simulink model "matched_filter_offset_estimation_correction"  (R2014b)
settings: Solver=FixedStepDiscrete  SolverMode=SingleTasking  StartTime=0.0  StopTime=run_time  RelTol=1e-3
PreLoadFcn:
  | %%%%%%%%%%%%%%%%%%%%%%%%%%%%%%%%%%%%%%%%%%%%%%%%%%%%%%%%%%%%%%%%%%%%%%%%%%%
  | % check to see if Simulink library folder is missing from the MATLAB path %
  | %%%%%%%%%%%%%%%%%%%%%%%%%%%%%%%%%%%%%%%%%%%%%%%%%%%%%%%%%%%%%%%%%%%%%%%%%%%
  | if isempty(strfind(path, 'rtlsdr_book_library'))
  | 
  |     % create error window
  |     fig_error = figure(...
  |         'Name', 'Error: RTL-SDR Book Library',...
  |         'Toolbar','none',...
  |         'MenuBar','none',...
  |         'NumberTitle','off',...
  |         'Resize','off',...
  |         'WindowStyle','modal');
  |     fig_error.Position(3) = 600;
  |     fig_error.Position(4) = 150;
  |     fig_axes = axes(...
  |         'Parent',fig_error,...
  |         'Position',[0,0,1,1],...
  |         'visible','off');
  |     % error message
  |     t_title = text(.05,.8,...
  |         'MISSING DIRECTORIES',...
  |         'FontSize',11.5);
  |     t_body = text(.075,.6,...
  |         [{'Simulink cannot find the  \it{<root>}\rm / \it{rtlsdr\_book\_library}\rm  folder in the \it{MATLAB Path}\rm.'},...
  |         {'Please set the MATLAB path following the instructions given in Exercise 2.4.'}],...
  |         'FontSize',10.5);
  |     % buttons
  |     btn_path = uicontrol(...
  |         'Parent',fig_error,...
  |         'String','Set Path Now',...
  |         'FontSize',10,...
  |         'Callback', 'pathtool; close(fig_error);',...
  |         'Position', [fig_error.Position(3)/2-210, 30, 200, 30]);
  |     btn_abort = uicontrol(...
  |         'Parent',fig_error,...
  |         'String','No thanks',...
  |         'FontSize',10,...
  |         'Callback', 'close(fig_error); abort=1;',...
  |         'Position', [fig_error.Position(3)/2+10, 30, 200, 30]);
  | 
  |     % pause to allow user to interact with error box
  |     uiwait(fig_error);
  | 
  |     % abort simulation
  |     try
  |         if abort==1
  |             set_param(gcs, 'SimulationCommand', 'stop');
  |         end
  |     end
  | 
  |     % if user has set path, allow diagram to be updated
  |     if ~exist('abort','var')
  |         % create error window
  |         fig_update = figure(...
  |             'Name', 'Update Diagram',...
  |             'Toolbar','none',...
  |             'MenuBar','none',...
  |             'NumberTitle','off',...
  |             'Resize','off');
  |         fig_update.Position(3) = 400;
  |         fig_update.Position(4) = 120;
  |         fig_axes = axes(...
  |             'Parent',fig_update,...
  |             'Position',[0,0,1,1],...
  |             'visible','off');
  |         % instruction message
  |         t_body = text(.075,.7,...
  |             'Once you have set the path, update the block diagram',...
  |             'FontSize',10.5);
  |         % button
  |         btn_update = uicontrol(...
  |             'Parent',fig_update,...
  |             'String','Update Block Diagram',...
  |             'FontSize',10,...
  |             'Callback', 'set_param(gcs,''SimulationCommand'',''update''); close(gcf)',...
  |             'Position', [fig_update.Position(3)/2-100, 30, 200, 30]);
  |     end
  | 
  |     % clear error components
  |     clear('fig_error','fig_update','fig_axes','t_title','t_body','btn_path','btn_abort','btn_update','abort');
  | 
  | end
  | %%%%%%%%%%%%%%%%%%%%%%%%%%%%%%%%%%%%%%%%%%%%%%%%%%%%%%%%%%%%%%%%%%%%%%%%%%%
  | 
  | 
  | % create default variable for running model
  | run_time = 7.3;
undefined symbols (not defined in the file): rec
libraries: simulink x5, rtlsdr_book_library x2, commutil2 x2, commdigbbndpm3 x2, dspmtrx3 x1
CloseFcn:
  | closefcn_model;
Description:
  | Software, Simulation Examples and Design Exercises Licence Agreement
  | 
  | This license agreement refers to the simulation examples, design exercises and files,
  | and associated software MATLAB and Simulink resources that accompany the book:
  | 
  |      Title: Software Defined Radio using MATLAB & Simulink and the RTL-SDR
  |      Published by Strathclyde Academic Media, 2015
  |      Authored by Robert W. Stewart, Kenneth W. Barlee, Dale S.W. Atkinson,
  |      and Louise H. Crockett
  | 
  | and made available as a download from, www.desktopSDR.com or variously acquired
  | by other means such as via USB storage, cloud storage, disk or any other electronic
  | or optical or magnetic storage mechanism. These files and associated software may
  | be used subject to the terms of agreement of the conditions below:
  | 
  |     Copyright © 2015 Robert W. Stewart, Kenneth W. Barlee, Dale S.W. Atkinson,
  |     and Louise H. Crockett
  |     All rights reserved.
  | 
  | Redistribution and use in source and binary forms, with or without modification, are
  | permitted provided that the following conditions are met:
  | 
  |    1.  Redistributions of source code must retain the above copyright notice, this list of
  |         conditions and the following disclaimer.
  | 
  |    2.  Redistributions in binary form must reproduce the above copyright notice, this
  |         list of conditions and the following disclaimer in the documentation and/or other
  |         materials provided with the distribution.
  | 
  |    3.  Neither the name of the copyright holder nor the names of its contributors may
  |         be used to endorse or promote products derived from this software without
  |         specific prior written permission.
  | 
  |    4.  In all cases, the software is, and all modifications and derivatives of the
  |         software shall be, licensed to you solely for use in conjunction with The
  |         MathWorks, Inc. products and service offerings.
  | 
  | THIS SOFTWARE IS PROVIDED BY THE COPYRIGHT HOLDERS AND CONTRIBUTORS
  | "AS IS" AND ANY EXPRESS OR IMPLIED WARRANTIES, INCLUDING, BUT NOT LIMITED
  | TO, THE IMPLIED WARRANTIES OF MERCHANTABILITY AND FITNESS FOR A
  | PARTICULAR PURPOSE ARE DISCLAIMED. IN NO EVENT SHALL THE COPYRIGHT
  | HOLDER OR CONTRIBUTORS BE LIABLE FOR ANY DIRECT, INDIRECT, INCIDENTAL,
  | SPECIAL, EXEMPLARY, OR CONSEQUENTIAL DAMAGES (INCLUDING, BUT NOT
  | LIMITED TO, PROCUREMENT OF SUBSTITUTE GOODS OR SERVICES; LOSS OF USE,
  | DATA, OR PROFITS; OR BUSINESS INTERRUPTION) HOWEVER CAUSED AND ON ANY
  | THEORY OF LIABILITY, WHETHER IN CONTRACT, STRICT LIABILITY, OR TORT
  | (INCLUDING NEGLIGENCE OR OTHERWISE) ARISING IN ANY WAY OUT OF THE USE
  | OF THIS SOFTWARE, EVEN IF ADVISED OF THE POSSIBILITY OF SUCH DAMAGE.
  | 
  | 
  | Audio Tracks used in Simulations Examples and Design Exercises
  | 
  | The music and vocal files used within the Examples files and software within the book
  | were variously written, arranged, performed, recorded and produced by Garrey Rice,
  | Adam Struth, Jamie Struth, Iain Thistlethwaite and also Marshall Craigmyle who
  | collectively, and individually where appropriate, assert and retain all of their copyright,
  | performance and artistic rights. Permission to use and reproduce this music is
  | granted for all purposes associated with MATLAB and Simulink software and the
  | simulation examples and design exercises files that accompany this book. Requests to
  | use the music for any other purpose should be directed to: info@desktopSDR.com.
  | For information on music track names, full credits, and links to the musicians please
  | refer to www.desktopSDR.com/more/audio.
settings Model: Creator=desktopSDR Team  LastModifiedBy=desktopSDR Team
settings DataIOCC: LimitDataPoints=off  SaveOutput=off  SignalLogging=off  SaveTime=off

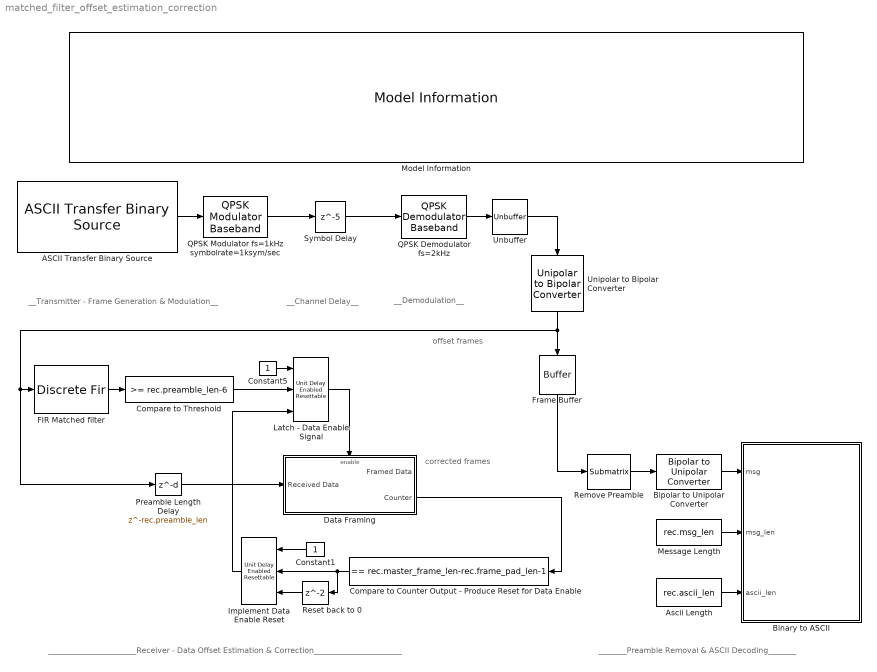
== system matched_filter_offset_estimation_correction ==
  note: corrected frames
  note: offset frames
  note: __Transmitter - Frame Generation & Modulation__
  note: __Channel Delay__
  note: __Demodulation__
  note: ______________________Receiver - Data Offset Estimation & Correction______________________
  note: _______Preamble Removal & ASCII Decoding_______
  "  ASCII Transfer Binary Source" : rtlsdr_book_library/Data Comms Sources and Sinks/  ASCII Transfer Binary Source  msg_tx=Hello World!  fs=2e3
  Ascii Length : Constant  Value=rec.ascii_len  VectorParams1D=off  OutDataTypeStr=single  FramePeriod=4096/240e3
  Binary to ASCII : MATLAB Function  TreatAsAtomicUnit=on
      mask init:
      | %% FIGURE SETUP        
      | %figure;
      | 
      | % resize
      | %window_x = 500;
      | %window_y = 500;
      | %window_width = 500;
      | %window_height = 110;
      | %set(gcf, 'Position', [window_x window_y window_width window_height]);
      | %set(gcf, 'menubar', 'none');
  Bipolar to Unipolar Converter : commutil2/Bipolar to Unipolar Converter  M=2  polarity=Positive  dataType=Inherit via internal rule
  Compare to Counter Output - Produce Reset for Data Enable : simulink/Logic and Bit Operations/Compare To Constant  relop===  const=rec.master_frame_len-rec.frame_pad_len-1  OutDataTypeStr=boolean
  Compare to Threshold : simulink/Logic and Bit Operations/Compare To Constant  relop=>=  const=rec.preamble_len-6  OutDataTypeStr=boolean
  Constant1 : Constant
  Constant5 : Constant
  Data Framing : Subsystem
  FIR Matched filter : DiscreteFir  Coefficients=rec.filter_coeff  InputProcessing=Columns as channels (frame based)
  Frame Buffer : Buffer  N=rec.master_frame_len  TreatMby1Signals=One channel
  Implement Data Enable Reset : simulink/Additional Math & Discrete/Additional Discrete/Unit Delay Enabled Resettable  vinit=0  tsamp=-1
  Latch - Data Enable Signal : simulink/Additional Math & Discrete/Additional Discrete/Unit Delay Enabled Resettable  vinit=0  tsamp=-1
  Message Length : Constant  Value=rec.msg_len  VectorParams1D=off  OutDataTypeStr=single  FramePeriod=-1
  Model Information : rtlsdr_book_library/Additional Tools/Model Information/Model Information
  Preamble Length Delay : Delay  DelayLength=rec.preamble_len  DelayLengthUpperLimit=10000  InitialCondition=1
  QPSK Demodulator fs=2kHz : commdigbbndpm3/QPSK Demodulator Baseband  Ph=pi/4  Dec=Gray  OutType=Bit  DecType=Hard decision  VarSource=Dialog  Variance=1  outDtype1=single  outDtype2=Inherit via internal rule  derotateFactorWordLen=16
  QPSK Modulator fs=1kHz symbolrate=1ksym/sec : commdigbbndpm3/QPSK Modulator Baseband  InType=Bit  Enc=Gray  Ph=pi/4  outDtype=single  outWordLen=16  outUDDataType=sfix(16)  outFracLenMode=Best precision  outFracLen=15
  Remove Preamble : dspmtrx3/Submatrix  RowSpan=Range of rows  RowStartMode=Index  RowStartIndex=rec.preamble_len+rec.preamble_pad_len+1  RowEndMode=Index  RowEndIndex=rec.master_frame_len-rec.frame_pad_len  ColSpan=One column  ColStartMode=First  ColStartIndex=1  ColEndMode=Last  ColEndIndex=1
  Reset back to 0 : Delay  DelayLengthUpperLimit=10000  InitialCondition=0
  Symbol Delay : Delay  DelayLength=5  InitialCondition=0  InputProcessing=Columns as channels (frame based)
  Unbuffer : Unbuffer  SampleBasedProcessing=Same as frame based
  Unipolar to Bipolar Converter : commutil2/Unipolar to Bipolar Converter  M=2  polarity=Positive  dataType=Inherit via internal rule
  wires:
  "  ASCII Transfer Binary Source"/1 -> QPSK Modulator fs=1kHz symbolrate=1ksym/sec/1
  Symbol Delay/1 -> QPSK Demodulator fs=2kHz/1
  Ascii Length/1 -> Binary to ASCII/3(ascii_len)
  Message Length/1 -> Binary to ASCII/2(msg_len)
  Bipolar to Unipolar Converter/1 -> Binary to ASCII/1(msg)
  QPSK Modulator fs=1kHz symbolrate=1ksym/sec/1 -> Symbol Delay/1
  QPSK Demodulator fs=2kHz/1 -> Unbuffer/1
  Remove Preamble/1 -> Bipolar to Unipolar Converter/1
  Unbuffer/1 -> Unipolar to Bipolar Converter/1
  Compare to Threshold/1 -> Latch - Data Enable Signal/2
  Constant5/1 -> Latch - Data Enable Signal/1
  Preamble Length Delay/1 -> Data Framing/1(Received Data)
  Data Framing/2(Counter) -> Compare to Counter Output - Produce Reset for Data Enable/1
  Compare to Counter Output - Produce Reset for Data Enable/1 -> Implement Data Enable Reset/2, Reset back to 0/1
  Constant1/1 -> Implement Data Enable Reset/1
  Reset back to 0/1 -> Implement Data Enable Reset/3
  Implement Data Enable Reset/1 -> Latch - Data Enable Signal/3
  Unipolar to Bipolar Converter/1 -> Preamble Length Delay/1, FIR Matched filter/1, Frame Buffer/1
  FIR Matched filter/1 -> Compare to Threshold/1
  Latch - Data Enable Signal/1 -> Data Framing/Enable
  Frame Buffer/1 -> Remove Preamble/1

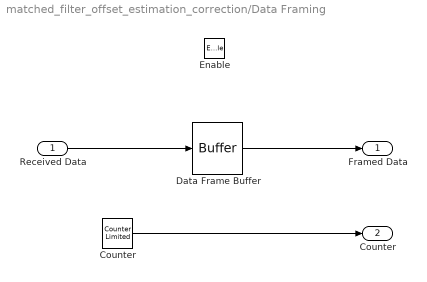
== system matched_filter_offset_estimation_correction/Data Framing ==
  Received Data : Inport
  Enable : EnablePort
  "Counter " : simulink/Sources/Counter Limited  uplimit=rec.master_frame_len-rec.frame_pad_len-1  tsamp=-1
  Data Frame Buffer : Buffer  N=rec.master_frame_len-rec.frame_pad_len  TreatMby1Signals=One channel
  Framed Data : Outport
  Counter : Outport  Port=2
  wires:
  Received Data/1 -> Data Frame Buffer/1
  Data Frame Buffer/1 -> Framed Data/1
  "Counter "/1 -> Counter/1

== matlab function matched_filter_offset_estimation_correction/Binary to ASCII ==
  data: msg input; msg_len input; ascii_len input
function msg_decoder(msg,msg_len,ascii_len)

% assert limits of msg_len for compiler
assert(msg_len>=1)
assert(msg_len<=2000)

% enable functions to be used by compiler
coder.extrinsic('uicontrol')
coder.extrinsic('disp')
coder.extrinsic('num2str')

% initialise output word with zeros
word = char(zeros(1,msg_len));

% convert ascii bits to ascii chars, save to string
for count = 1:1:msg_len
    char_bin = msg((((count-1)*ascii_len)+1):ascii_len*count)';
    word(count) = char(bi2de(char_bin,'left-msb'));
end
disp(word);    
end
